simulink model "Test_Freq_Resp_3"  (Simulink 8.3)
settings: Solver=ode4  StartTime=0.0  StopTime=N-1  FixedStep=T  RelTol=1e-3
values from neighbouring files (symbols this model uses):
  A = 1    [Start_Up.m]
  N = 256    [Start_Up.m]
  T = .001    (= 0.001)    [Start_Up.m]
  w_end = 1.5/T    (= 1500)    [Start_Up.m]
  w_start = .1/T    (= 100)    [Start_Up.m]
libraries: cstblocks x2
settings Model: Creator=baqumau  LastModifiedBy=baqumau
settings DataIOCC: SignalLoggingSaveFormat=Dataset
settings DebuggingCC: UnderspecifiedInitializationDetection=Simplified  StateNameClashWarn=none
settings GRTTargetCC: CombineOutputUpdateFcns=on  GRTInterface=off

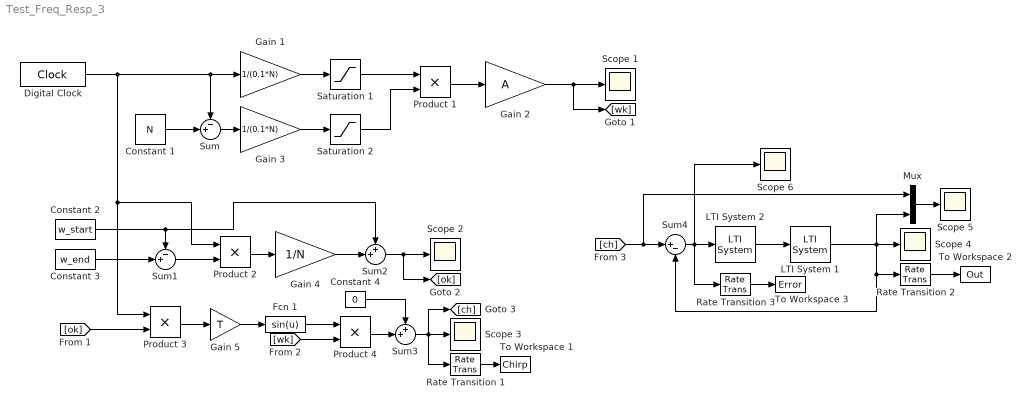
== system Test_Freq_Resp_3 ==
  Constant 1 : Constant  Value=N
  Constant 2 : Constant  Value=w_start
  Constant 3 : Constant  Value=w_end
  Constant 4 : Constant  Value=0
  Digital Clock : DigitalClock  SampleTime=T
  Fcn 1 : Fcn  Expr=sin(u)
  Gain 1 : Gain  Gain=1/(0.1*N)
  Gain 2 : Gain  Gain=A
  Gain 3 : Gain  Gain=1/(0.1*N)
  Gain 4 : Gain  Gain=1/N
  Gain 5 : Gain  Gain=T
  LTI System 1 : cstblocks/LTI System  sys=G  IC=[]
  LTI System 2 : cstblocks/LTI System  sys=K  IC=[]
  Mux : Mux  Inputs=2
  Product {1..4} (4 alike) : Product
  Rate Transition 1 : RateTransition  OutPortSampleTime=Ts
  Rate Transition 2 : RateTransition  OutPortSampleTime=Ts
  Rate Transition 3 : RateTransition  OutPortSampleTime=Ts
  Saturation 1 : Saturate  UpperLimit=1  LowerLimit=-1
  Saturation 2 : Saturate  UpperLimit=1  LowerLimit=-1
  Scope {1..6} (6 alike) : Scope
      Scope 3 settings: SaveName=ScopeData2
      Scope 4 settings: SaveName=ScopeData3
      Scope 5 settings: SaveName=ScopeData4
      Scope 6 settings: SaveName=ScopeData5
  Sum : Sum  Inputs=-+|
  Sum1 : Sum  Inputs=-+|
  Sum2 : Sum  Inputs=++|
  Sum3 : Sum  Inputs=++|
  Sum4 : Sum  Inputs=|+-
  To Workspace 1 : ToWorkspace  VariableName=Chirp  SaveFormat=Structure With Time  SampleTime=-1
  To Workspace 2 : ToWorkspace  VariableName=Out  SaveFormat=Structure With Time  SampleTime=-1
  To Workspace 3 : ToWorkspace  VariableName=Error  SaveFormat=Structure With Time  SampleTime=-1
  wires:
  Gain 1/1 -> Saturation 1/1
  Saturation 1/1 -> Product 1/1
  Digital Clock/1 -> Product 3/1, Product 2/1, Gain 1/1, Sum/1
  Sum/1 -> Gain 3/1
  Constant 1/1 -> Sum/2
  Gain 3/1 -> Saturation 2/1
  Saturation 2/1 -> Product 1/2
  Product 1/1 -> Gain 2/1
  Gain 2/1 -> [wk], Scope 1/1
  Constant 2/1 -> Sum2/1, Sum1/1
  Constant 3/1 -> Sum1/2
  Sum1/1 -> Product 2/2
  Product 2/1 -> Gain 4/1
  Gain 4/1 -> Sum2/2
  Sum2/1 -> [ok], Scope 2/1
  [ok] -> Product 3/2
  Product 3/1 -> Gain 5/1
  Gain 5/1 -> Fcn 1/1
  Fcn 1/1 -> Product 4/1
  [wk] -> Product 4/2
  Product 4/1 -> Sum3/2
  Sum3/1 -> [ch], Rate Transition 1/1, Scope 3/1
  LTI System 1/1 -> Mux/2, Rate Transition 2/1, Sum4/2, Scope 4/1
  Mux/1 -> Scope 5/1
  Rate Transition 2/1 -> To Workspace 2/1
  Rate Transition 1/1 -> To Workspace 1/1
  Constant 4/1 -> Sum3/1
  [ch] -> Sum4/1, Mux/1
  Sum4/1 -> Scope 6/1, Rate Transition 3/1, LTI System 2/1
  LTI System 2/1 -> LTI System 1/1
  Rate Transition 3/1 -> To Workspace 3/1
